simulink model "DirectDriveSubsystem"  (R2022b)
settings: Solver=VariableStepAuto  StartTime=0.0  StopTime=10.0  RelTol=1e-3
values from neighbouring files (symbols this model uses):
  generatorJ = 20    [wecSimInputFile.m]
  generatorR = .483    (= 0.483)    [wecSimInputFile.m]
  Kt = 7.186    [wecSimInputFile.m]
  shaftMechDamping = 1    [wecSimInputFile.m]
  tcControl = generatorL/generatorR    (= 0.0108136645963)    [wecSimInputFile.m]
undefined symbols (not defined in the file or in its folder): magnitude, pinionRad, PinionRad
settings Model: Creator=dforbus  LastModifiedBy=jtgrasb

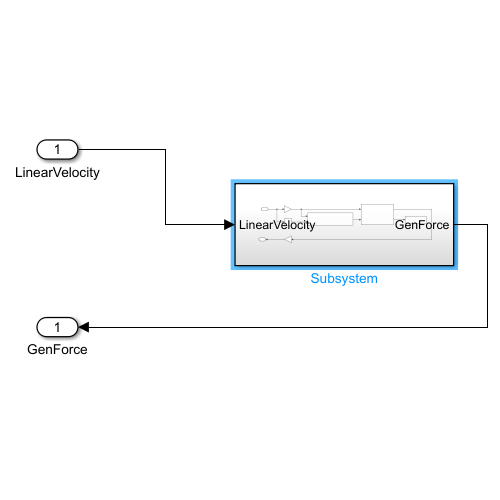
[thumbnail: Simulink's stored preview of the top-level diagram]
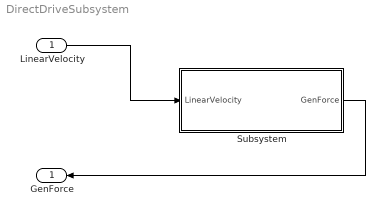
== system DirectDriveSubsystem ==
  LinearVelocity : Inport
  Subsystem : Subsystem
  GenForce : Outport
  wires:
  LinearVelocity/1 -> Subsystem/1(LinearVelocity)
  Subsystem/1(GenForce) -> GenForce/1

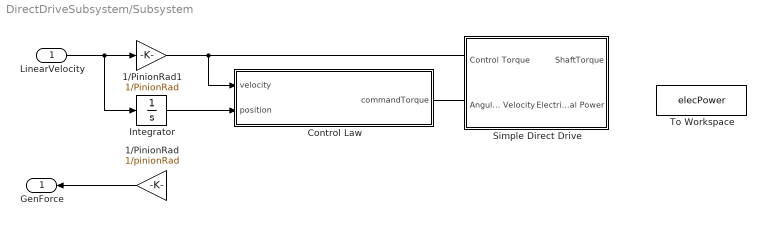
== system DirectDriveSubsystem/Subsystem ==
  LinearVelocity : Inport
  1/PinionRad : Gain  Gain=1/pinionRad
  1/PinionRad1 : Gain  Gain=1/PinionRad
  Control Law : MATLAB Function  TreatAsAtomicUnit=on
  Integrator : Integrator
  Simple Direct Drive : Subsystem  TreatAsAtomicUnit=on
  To Workspace : ToWorkspace  VariableName=elecPower  SaveFormat=Timeseries  SampleTime=-1
  GenForce : Outport
  wires:
  Control Law/1(commandTorque) -> ?
  1/PinionRad1/1 -> Control Law/1(velocity)
  ? -> To Workspace/1
  1/PinionRad/1 -> GenForce/1
  LinearVelocity/1 -> Integrator/1, 1/PinionRad1/1
  ? -> 1/PinionRad/1
  Integrator/1 -> Control Law/2(position)

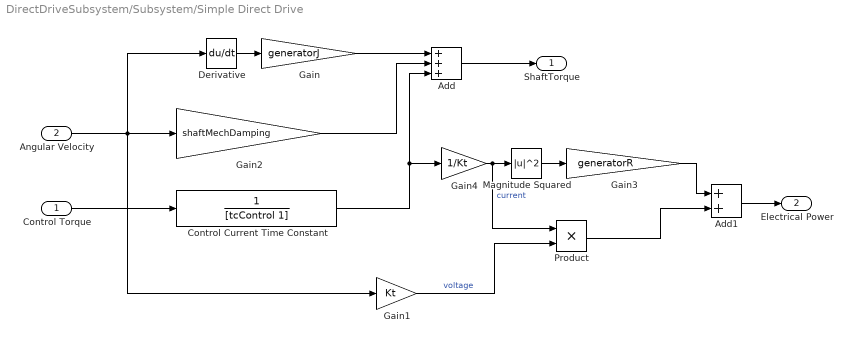
== system DirectDriveSubsystem/Subsystem/Simple Direct Drive ==
  Control Torque : Inport
  Angular Velocity : Inport  Port=2
  Add : Sum  Inputs=+++
  Add1 : Sum
  Control Current Time Constant : TransferFcn  Denominator=[tcControl 1]
  Derivative : Derivative  CoefficientInTFapproximation=1000*2*pi
  Gain : Gain  Gain=generatorJ
  Gain1 : Gain  Gain=Kt
  Gain2 : Gain  Gain=shaftMechDamping
  Gain3 : Gain  Gain=generatorR
  Gain4 : Gain  Gain=1/Kt
  Magnitude Squared : Math  Operator=magnitude^2
  Product : Product
  ShaftTorque : Outport
  Electrical Power : Outport  Port=2
  wires:
  Gain/1 -> Add/1
  Control Torque/1 -> Control Current Time Constant/1
  Gain1/1 -> Product/2  "voltage"
  Control Current Time Constant/1 -> Add/3, Gain4/1
  Add/1 -> ShaftTorque/1
  Gain2/1 -> Add/2
  Product/1 -> Add1/2
  Add1/1 -> Electrical Power/1
  Gain4/1 -> Product/1, Magnitude Squared/1  "current"
  Angular Velocity/1 -> Gain1/1, Gain2/1, Derivative/1
  Derivative/1 -> Gain/1
  Magnitude Squared/1 -> Gain3/1
  Gain3/1 -> Add1/1

== matlab function DirectDriveSubsystem/Subsystem/Control Law ==
  data: velocity input; commandTorque output; position input
function commandTorque = PIControl(velocity,position)

commandTorque = KI*position + KP*velocity;

end
